simulink model "CT_UDE"  (R2021a)
settings: Solver=ode4  StartTime=0.0  StopTime=tstop  FixedStep=tstep  RelTol=1e-3
values from neighbouring files (symbols this model uses):
  eic = xic - xmic    [data.m]
  K = place(A_n, B_n, eig(A_m))    [data.m]
  xic = zeros(4, 1)    [data.m]
  xmic = zeros(4, 1)    [data.m]
settings Model: Creator=Ram Padmanabhan  LastModifiedBy=Ram Padmanabhan
settings SolverCC: AlgebraicLoopSolver=TrustRegion
settings DataIOCC: SaveOutput=off  SignalLogging=off  DSMLogging=off  SaveTime=off  ReturnWorkspaceOutputs=off
settings DebuggingCC: SFMachineParentedDataDiag=warning

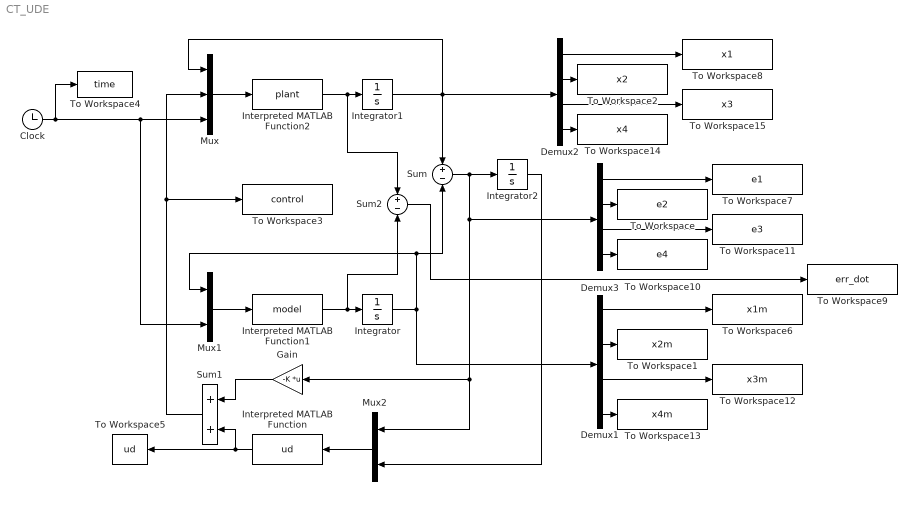
== system CT_UDE ==
  Clock : Clock
  Demux1 : Demux
  Demux2 : Demux
  Demux3 : Demux
  Gain : Gain  Gain=-K  Multiplication=Matrix(K*u)
  Integrator : Integrator  InitialCondition=xmic
  Integrator1 : Integrator  InitialCondition=xic
  Integrator2 : Integrator  InitialCondition=eic
  Interpreted MATLAB Function : MATLABFcn  MATLABFcn=ud  OutputDimensions=2
  Interpreted MATLAB Function1 : MATLABFcn  MATLABFcn=model  OutputDimensions=4
  Interpreted MATLAB Function2 : MATLABFcn  MATLABFcn=plant  OutputDimensions=4
  Mux : Mux  Inputs=3
  Mux1 : Mux  Inputs=2
  Mux2 : Mux  Inputs=2
  Sum : Sum  Inputs=+-
  Sum1 : Sum
  Sum2 : Sum  Inputs=+-
  To Workspace : ToWorkspace  VariableName=e2  SampleTime=-1
  To Workspace1 : ToWorkspace  VariableName=x2m  SampleTime=-1
  To Workspace10 : ToWorkspace  VariableName=e4  SampleTime=-1
  To Workspace11 : ToWorkspace  VariableName=e3  SampleTime=-1
  To Workspace12 : ToWorkspace  VariableName=x3m  SampleTime=-1
  To Workspace13 : ToWorkspace  VariableName=x4m  SampleTime=-1
  To Workspace14 : ToWorkspace  VariableName=x4  SampleTime=-1
  To Workspace15 : ToWorkspace  VariableName=x3  SampleTime=-1
  To Workspace2 : ToWorkspace  VariableName=x2  SampleTime=-1
  To Workspace3 : ToWorkspace  VariableName=control  SampleTime=-1
  To Workspace4 : ToWorkspace  VariableName=time  SampleTime=-1
  To Workspace5 : ToWorkspace  VariableName=ud  SampleTime=-1
  To Workspace6 : ToWorkspace  VariableName=x1m  SampleTime=-1
  To Workspace7 : ToWorkspace  VariableName=e1  SampleTime=-1
  To Workspace8 : ToWorkspace  VariableName=x1  SampleTime=-1
  To Workspace9 : ToWorkspace  VariableName=err_dot  SampleTime=-1
  wires:
  Interpreted MATLAB Function2/1 -> Sum2/1, Integrator1/1
  Interpreted MATLAB Function1/1 -> Sum2/2, Integrator/1
  Mux/1 -> Interpreted MATLAB Function2/1
  Integrator1/1 -> Mux/1, Demux2/1, Sum/1
  Clock/1 -> Mux/3, Mux1/2, To Workspace4/1
  Mux1/1 -> Interpreted MATLAB Function1/1
  Integrator/1 -> Sum/2, Mux1/1, Demux1/1
  Sum/1 -> Integrator2/1, Gain/1, Mux2/1, Demux3/1
  Mux2/1 -> Interpreted MATLAB Function/1
  Integrator2/1 -> Mux2/2
  Gain/1 -> Sum1/1
  Interpreted MATLAB Function/1 -> To Workspace5/1, Sum1/2
  Sum1/1 -> To Workspace3/1, Mux/2
  Demux3/1 -> To Workspace7/1
  Demux3/2 -> To Workspace/1
  Demux1/1 -> To Workspace6/1
  Demux1/2 -> To Workspace1/1
  Sum2/1 -> To Workspace9/1
  Demux3/4 -> To Workspace10/1
  Demux3/3 -> To Workspace11/1
  Demux1/4 -> To Workspace13/1
  Demux1/3 -> To Workspace12/1
  Demux2/2 -> To Workspace2/1
  Demux2/3 -> To Workspace15/1
  Demux2/4 -> To Workspace14/1
  Demux2/1 -> To Workspace8/1
